simulink model "SignalTest"  (R2024a)
settings: Solver=VariableStepAuto  StartTime=0.0  StopTime=10.0  RelTol=1e-3
libraries: simulink x1
settings Model: Creator=jherr  LastModifiedBy=jherr

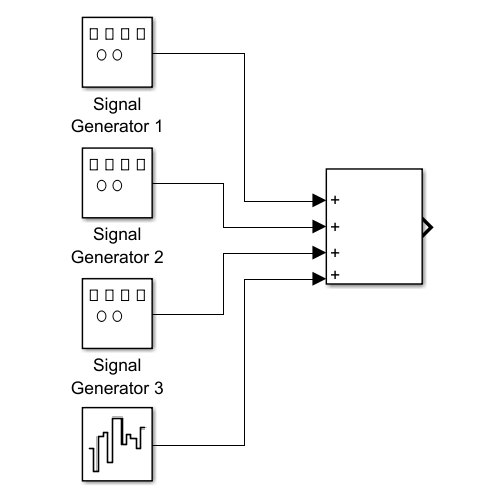
[thumbnail: Simulink's stored preview of the top-level diagram]
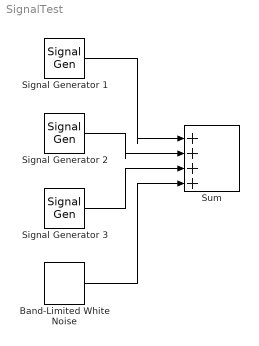
== system SignalTest ==
  Band-Limited White Noise : simulink/Sources/Band-Limited White Noise  Cov=[4]  Ts=0.001  seed=[23341]
  Signal Generator 1 : SignalGenerator  Frequency=40*pi  Units=rad/sec
  Signal Generator 2 : SignalGenerator  Frequency=200*pi  Units=rad/sec
  Signal Generator 3 : SignalGenerator  Frequency=400*pi  Units=rad/sec
  Sum : Sum  Inputs=|++++
  wires:
  Signal Generator 1/1 -> Sum/1
  Signal Generator 2/1 -> Sum/2
  Signal Generator 3/1 -> Sum/3
  Band-Limited White Noise/1 -> Sum/4
